simulink library "library_ALICAT_CODA_RW"  (R2024b)
settings: Solver=VariableStepAuto  StartTime=0.0  StopTime=10.0  RelTol=1e-3
undefined symbols (not defined in the file or in its folder): Controller
settings Model: Creator=GavinWilliamson  LastModifiedBy=GavinWilliamson

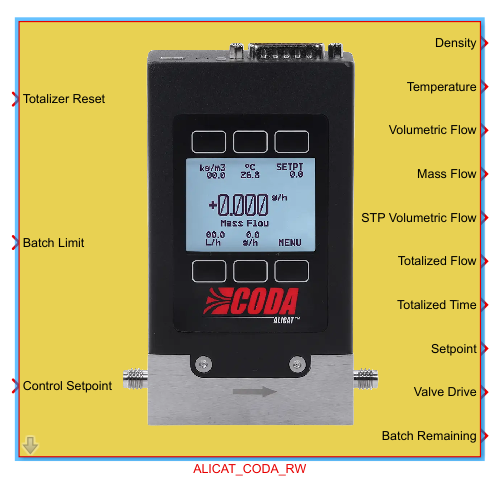
[thumbnail: Simulink's stored preview of the top-level diagram]
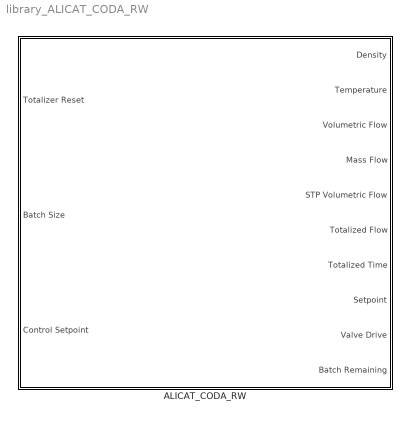
== system library_ALICAT_CODA_RW ==
  ALICAT_CODA_RW : Subsystem  mask{Port="COM4", Device_Name='A', gs_type=Hydrogen, dv_typ=Controller, totlzer_typ=Mass Flow Rate, vlvDR_sw=on, cntrl_sw=on, batch_sw=on}
      mask prompts: Device_Name "Device Identifier"; gs_type "Gas Type"; dv_typ "Device Type"; totlzer_typ "Totalizer Variable"; vlvDR_sw "Enable Valve Drive Recording"; cntrl_sw "Enable ALICAT Controller"; batch_sw "Enable Batching"
      mask help: Default Mask
      mask Help: web(which('help_ALICAT_CODA_RW.html'), '-helpbrowser')
      mask TypeOptions Port:
      | Level-2 MATLAB
      | S-Function/Port
      mask TypeOptions Device_Name:
      | Level-2 MATLAB
      | S-Function/Device_Name
      mask TypeOptions gs_type:
      | Level-2 MATLAB
      | S-Function/gs_type
      mask TypeOptions dv_typ:
      | Level-2 MATLAB
      | S-Function/dv_typ
      mask TypeOptions totlzer_typ:
      | Level-2 MATLAB
      | S-Function/totlzer_typ
      mask TypeOptions vlvDR_sw:
      | Level-2 MATLAB
      | S-Function/vlvDR_sw
      mask TypeOptions cntrl_sw:
      | Level-2 MATLAB
      | S-Function/cntrl_sw
      mask TypeOptions batch_sw:
      | Level-2 MATLAB
      | S-Function/batch_sw
      mask DialogControl Container3 Prompt: General
      mask DialogControl DescGroupVar Prompt: ALICAT_CODA_RW
      mask DialogControl DescTextVar Prompt: Block controls and reads an ALICAT CODA devices over serial communication. Labels on the ports on the block will disappear if there are not valid for the configuration selected. To see all port labels you can look under the mask of this block.
      mask DialogControl Container5 Prompt: Communication Parameters
      mask DialogControl Container6 Prompt: Data Logging Options
      mask DialogControl Container7 Prompt: Control Options
      mask DialogControl Container4 Prompt: Instructions
      mask DialogControl Container8 Prompt: Inputs
      mask DialogControl Control2 Prompt: Totalizer Reset: Input should be a constant block that is set to 0. A push button should be linked to the block to change the value to 1 when pushed. When the button is pushed the totalizer will then be reset.
      mask DialogControl Control3 Prompt: Batch Limit: The input for totalizer limit will only be written to the device if the totalizer and batching are enabled in the register parameters.
      mask DialogControl Control4 Prompt: Control Setpoint: The for setting the setpoint of the device if "Enable ALICAT Controller" is checked. The control loop variable cannot be chosen using this block and should be selected by communicating with the device directly or thorugh the FlowVision software before the simulaiton is run.
      mask DialogControl Container11 Prompt: Register Parameters
      mask DialogControl Container9 Prompt: Communication Parameters
      mask DialogControl Control5 Prompt: Port: Communication port that ALICAT is connected to [string]
      mask DialogControl Control6 Prompt: Device Identifier: Unit ID of ALICAT [char]
      mask DialogControl Container10 Prompt: Gas Type
      mask DialogControl Control7 Prompt: Process gas flowing through ALICAT
      mask DialogControl Container12 Prompt: Device Type
      mask DialogControl Control8 Prompt: Select whether the ALICAT that is connected to the COM Port is a controller or meter. This is important to ensure invalid commands are not sent to the device, and to ensure that the outputted data is in the expected format.
      mask DialogControl Container13 Prompt: Data Logging Options
      mask DialogControl Control9 Prompt: Totalizer Variable: Select wether the totalizer uses mass flow rate or volumetric flow rate.
      mask DialogControl Control10 Prompt: Enable Valve Drive Recording: This will set the valve drive position to be outputted by an ALICAT controller.
      mask DialogControl Container14 Prompt: Control Options
      mask DialogControl Control11 Prompt: Enable ALICAT Controller: This allows an ALICAT controller to be controlled through Simulink. If unchecked, Simulink will just configure the data logging option parameters and read the device outputs.
      mask DialogControl Control12 Prompt: Enable Batching: This enables the batching on the ALICAT and enables the batch limit to be updated while the model is running.
      mask Display:
      | image('coda-display-meter-solo-prod.png',[10,0,10,0,100,100]);
      | 
      | %input ports
      | port_label('input', 1, 'Totalizer Reset');
      | if strcmp(get_param(gcb,'batch_sw'),'on')
      |     port_label('input', 2, 'Batch Limit');
      | end
      | if strcmp(get_param(gcb,'cntrl_sw'),'on')
      |     port_label('input', 3, 'Control Setpoint');
      | end
      | 
      | %output ports
      | port_label('output', 1, 'Density');
      | port_label('output', 2, 'Temperature');
      | port_label('output', 3, 'Volumetric Flow');
      | port_label('output', 4, 'Mass Flow');
      | port_label('output', 5, 'STP Volumetric Flow');
      | port_label('output', 6, 'Totalized Flow');
      | port_label('output', 7, 'Totalized Time');
      | if strcmp(get_param(gcb,'dv_typ'),'Controller')
      |     port_label('output', 8, 'Setpoint');
      | end
      | if strcmp(get_param(gcb,'vlvDr_sw'),'on')
      |     port_label('output', 9, 'Valve Drive');
      | end
      | if strcmp(get_param(gcb,'batch_sw'),'on')
      |     port_label('output', 10, 'Batch Remaining');
      | end

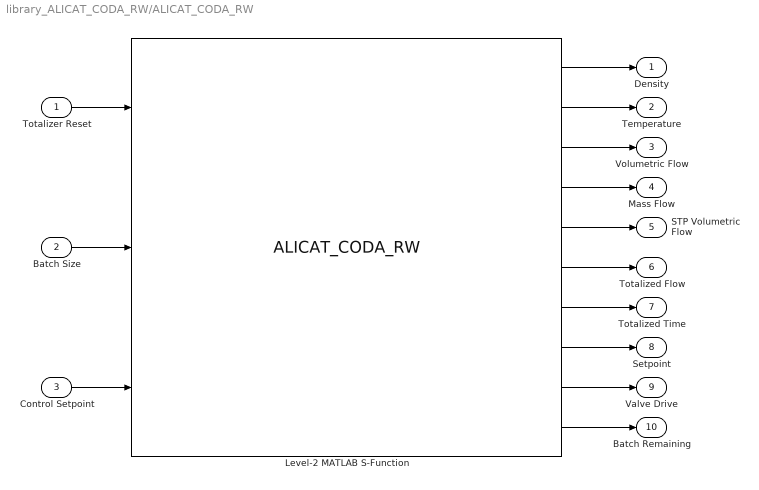
== system library_ALICAT_CODA_RW/ALICAT_CODA_RW ==
  Totalizer Reset : Inport
  Batch Size : Inport  Port=2
  Control Setpoint : Inport  Port=3
  Level-2 MATLAB S-Function : M-S-Function  FunctionName=ALICAT_CODA_RW  Parameters=Port, Device_Name, gs_type, batch_sw, contrl_typ, cntrl_sw, dv_typ,totlzer_typ,vlvDR_sw  mask{Port=Port, Device_Name=Device_Name, gs_type=Hydrogen, dv_typ=Controller, totlzer_typ=Mass Flow Rate, vlvDR_sw=on, cntrl_sw=on, contrl_typ=Mass Flow, batch_sw=on}
      mask prompts: Device_Name "Device Identifier"; gs_type "Gas Type"; dv_typ "Device Type"; totlzer_typ "Totalizer Variable"; vlvDR_sw "Enable Valve Drive Recording"; cntrl_sw "Enable ALICAT Controller"; contrl_typ "Setpoint Variable"; batch_sw "Enable Batching"
      mask TypeOptions gs_type: Hydrogen | Nitrogen | Air
      mask TypeOptions dv_typ: Controller | Meter
      mask TypeOptions totlzer_typ: Mass Flow Rate | Volumetric Flow Rate
      mask TypeOptions contrl_typ: Mass Flow | Volumetric Flow | Standardized Volumetric Flow
      mask DialogControl DescGroupVar Prompt: ALICAT__CODA_RW
      mask DialogControl DescTextVar Prompt: *See mask of subsystem
      mask DialogControl Container4 Prompt: Connection Parameters
      mask DialogControl Container5 Prompt: Data Logging Options
      mask DialogControl Container6 Prompt: Control Options
      mask Display:
      | image('coda-display-meter-solo-prod.png',[0,0,0,0,100,100]);
      | 
      | 
      | port_label('input', 1, 'Totalizer Reset');
      | port_label('input', 2, 'Batch Size');
      | port_label('input', 3, 'Control Setpoint');
      | 
      | port_label('output', 1, 'Density');
      | port_label('output', 2, 'Temperature');
      | port_label('output', 3, 'Volumetric Flow');
      | port_label('output', 4, 'Mass Flow');
      | port_label('output', 5, 'STP Volumetric Flow');
      | port_label('output', 6, 'Totalized Flow');
      | port_label('output', 7, 'Totalized Time');
      | port_label('output', 8, 'Setpoint');
      | port_label('output', 9, 'Valve Drive');
      | port_label('output', 10, 'Batch Remaining');
  Density : Outport
  Temperature : Outport  Port=2
  Volumetric Flow : Outport  Port=3
  Mass Flow : Outport  Port=4
  STP Volumetric Flow : Outport  Port=5
  Totalized Flow : Outport  Port=6
  Totalized Time : Outport  Port=7
  Setpoint : Outport  Port=8
  Valve Drive : Outport  Port=9
  Batch Remaining : Outport  Port=10
  wires:
  Level-2 MATLAB S-Function/2 -> Temperature/1
  Level-2 MATLAB S-Function/1 -> Density/1
  Control Setpoint/1 -> Level-2 MATLAB S-Function/3
  Level-2 MATLAB S-Function/3 -> Volumetric Flow/1
  Level-2 MATLAB S-Function/4 -> Mass Flow/1
  Level-2 MATLAB S-Function/5 -> STP Volumetric Flow/1
  Level-2 MATLAB S-Function/6 -> Totalized Flow/1
  Batch Size/1 -> Level-2 MATLAB S-Function/2
  Level-2 MATLAB S-Function/7 -> Totalized Time/1
  Totalizer Reset/1 -> Level-2 MATLAB S-Function/1
  Level-2 MATLAB S-Function/8 -> Setpoint/1
  Level-2 MATLAB S-Function/9 -> Valve Drive/1
  Level-2 MATLAB S-Function/10 -> Batch Remaining/1
